simulink model "Channel_Picking_Experiment"  (R2023a)
settings: Solver=ode23tb  StartTime=0.0  StopTime=0.5  RelTol=1e-3
libraries: dspindex x5, dspsnks4 x1, dspstat3 x1
settings Model: Creator=zacha  LastModifiedBy=zacha
settings DebuggingCC: UnconnectedInputMsg=warning  UnconnectedOutputMsg=warning  UnconnectedLineMsg=warning
settings ModelReferenceCC: EnableRefExpFcnMdlSchedulingChecks=on
settings RTWCC: DLArmComputeVersion=19.05

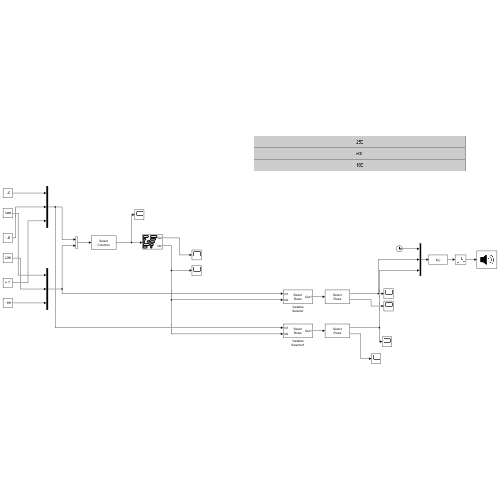
[thumbnail: Simulink's stored preview of the top-level diagram]
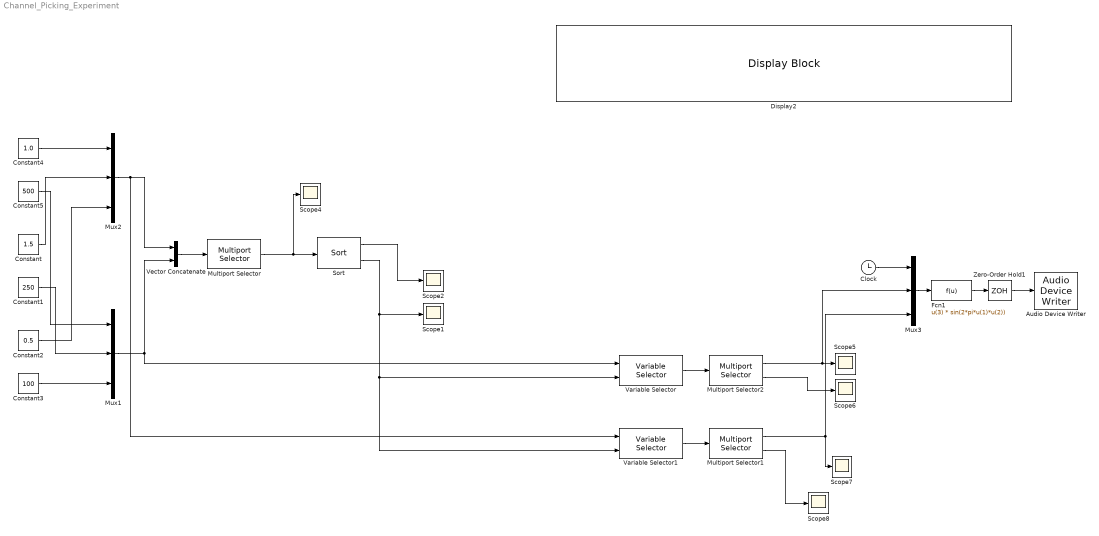
== system Channel_Picking_Experiment ==
  Audio Device Writer : dspsnks4/Audio Device Writer  Driver=DirectSound  Device=Default  InheritSampleRate=on  SampleRate=44100  BitDepth=16-bit integer  BufferSize=4096  NumBuffers=10  DefaultOutputChannelMapping=on  OutputChannelMapping=1:2  OutputNumUnderrunSamples=off  DriverIdx=1  DeviceWarnFlag=''
  Clock : Clock
  Constant : Constant  Value=1.5
  Constant1 : Constant  Value=250
  Constant2 : Constant  Value=0.5
  Constant3 : Constant  Value=100
  Constant4 : Constant  Value=1.0
  Constant5 : Constant  Value=500
  Display2 : DisplayBlock  LabelPosition=Hide  Transparency=1
  Fcn1 : Fcn  Expr=u(3) * sin(2*pi*u(1)*u(2))
  Multiport Selector : dspindex/Multiport Selector  rowsOrCols=Columns  idxCellArray={ 1 }  idxErrMode=Generate Error
  Multiport Selector1 : dspindex/Multiport Selector  rowsOrCols=Rows  idxCellArray={ 1, 2 }  idxErrMode=Clip Index
  Multiport Selector2 : dspindex/Multiport Selector  rowsOrCols=Rows  idxCellArray={ 1, 2 }  idxErrMode=Clip Index
  Mux1 : Mux  Inputs=3
  Mux2 : Mux  Inputs=3
  Mux3 : Mux  Inputs=3
  Scope{1..2,4..8} (7 alike) : Scope
  Sort : dspstat3/Sort  otype=Value and Index  dir=Descending  sortAlg=Quick sort  roundingMode=Floor  overflowMode=off  accumDataTypeStr=Inherit: Same as product output  accumLastDataTypeStr=Inherit: Same as product output
  Variable Selector : dspindex/Variable Selector  NumInputs=1  rowsOrCols=Rows  IdxMode=Variable  Elements=[1 3]  ZerOneIdxMode=One-based  errmode=Clip Index  FillMode=on  FillValues=0
      settings: LibrarySourceBlock=|
      | dsphdlsupportsigmgmt/Variable
      | Selector
  Variable Selector1 : dspindex/Variable Selector  NumInputs=1  rowsOrCols=Rows  IdxMode=Variable  Elements=[1 3]  ZerOneIdxMode=One-based  errmode=Clip Index  FillMode=on  FillValues=0
      settings: LibrarySourceBlock=|
      | dsphdlsupportsigmgmt/Variable
      | Selector
  Vector Concatenate : Concatenate  Mode=Multidimensional array  ConcatenateDimension=2
  Zero-Order Hold1 : ZeroOrderHold  SampleTime=1/8000
  wires:
  Multiport Selector/1 -> Sort/1, Scope4/1
  Sort/1 -> Scope2/1
  Vector Concatenate/1 -> Multiport Selector/1
  Sort/2 -> Variable Selector1/2, Variable Selector/2, Scope1/1
  Constant4/1 -> Mux2/1
  Constant/1 -> Mux2/2
  Constant2/1 -> Mux2/3
  Constant5/1 -> Mux1/1
  Constant1/1 -> Mux1/2
  Constant3/1 -> Mux1/3
  Mux2/1 -> Variable Selector1/1, Vector Concatenate/1
  Mux1/1 -> Vector Concatenate/2, Variable Selector/1
  Variable Selector/1 -> Multiport Selector2/1
  Multiport Selector2/1 -> Mux3/2, Scope5/1
  Multiport Selector2/2 -> Scope6/1
  Variable Selector1/1 -> Multiport Selector1/1
  Multiport Selector1/2 -> Scope8/1
  Mux3/1 -> Fcn1/1
  Clock/1 -> Mux3/1
  Multiport Selector1/1 -> Mux3/3, Scope7/1
  Fcn1/1 -> Zero-Order Hold1/1
  Zero-Order Hold1/1 -> Audio Device Writer/1
